simulink model "passive cell balancing"  (R2022a)
settings: Solver=VariableStepAuto  StartTime=0.0  StopTime=500  RelTol=1e-3
undefined symbols (not defined in the file): Ion, Lithium
libraries: spsIGBTLib x6, spsBatteryLib x4, spsSeriesRLCBranchLib x4, spsDCVoltageSourceLib x1, spsGroundLib x1, spsSeriesRLCLoadLib x1, spspowerguiLib x1
settings Model: Creator=my pc  LastModifiedBy=my pc

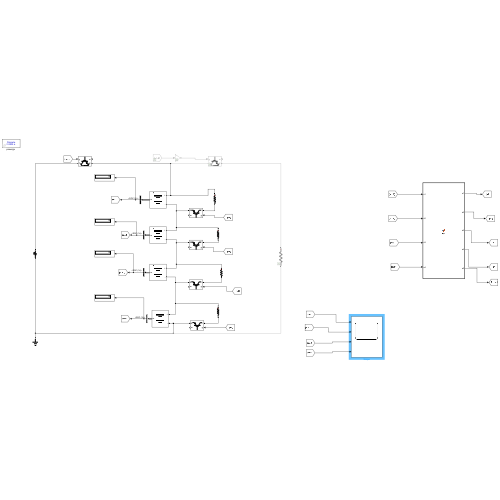
[thumbnail: Simulink's stored preview of the top-level diagram]
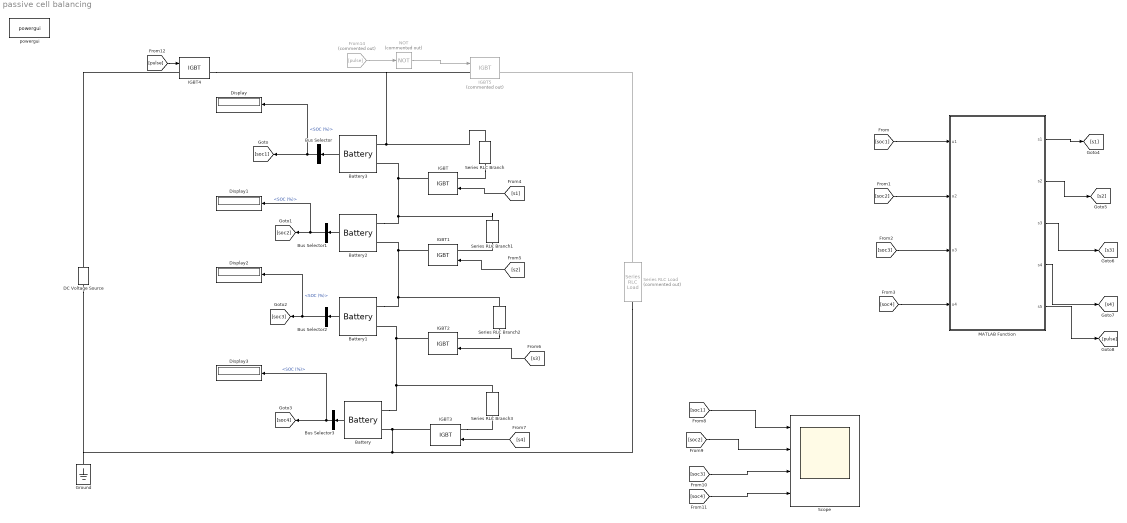
== system passive cell balancing ==
  Battery : spsBatteryLib/Battery  BatType=Lithium-Ion  ShowTempParam=off  ThermalPreset=no  ShowAgeParam=off  NomV=7.2  NomQ=5.4  SOC=19  Batt_Tr=30  PresetModel=on  MaxQ=5.4  MinV=5.4  FullV=8.3807  Dis_rate=2.3478  R=0.013333  Normal_OP=4.8835  expZone="[7.7788      0.2653]"  current=[6.5 13 32.5]  Units=Time  Tci=20  NomT=20  T2=-30  MaxQ2=4.8  FullV2=7.1  Normal_OP2=5.655  expZone2="[6.58           1]"  Rca=0.6  ti=2000  Dp=0  Neq0=0  Tsim=1e6  Ta1=25  Qeol=5.4*0.9  Reol=0.013333*1.2  Char_age=[2.3478, 3]  Dis_age=[2.3478, 10]  N1=1500  N2=10500  N3=1000  N4=1400  Ta2=45  N5=950
  Battery1 : spsBatteryLib/Battery  BatType=Lithium-Ion  ShowTempParam=off  ThermalPreset=no  ShowAgeParam=off  NomV=7.2  NomQ=5.4  SOC=21  Batt_Tr=30  PresetModel=on  MaxQ=5.4  MinV=5.4  FullV=8.3807  Dis_rate=2.3478  R=0.013333  Normal_OP=4.8835  expZone="[7.7788      0.2653]"  current=[6.5 13 32.5]  Units=Time  Tci=20  NomT=20  T2=-30  MaxQ2=4.8  FullV2=7.1  Normal_OP2=5.655  expZone2="[6.58           1]"  Rca=0.6  ti=2000  Dp=0  Neq0=0  Tsim=1e6  Ta1=25  Qeol=5.4*0.9  Reol=0.013333*1.2  Char_age=[2.3478, 3]  Dis_age=[2.3478, 10]  N1=1500  N2=10500  N3=1000  N4=1400  Ta2=45  N5=950
  Battery2 : spsBatteryLib/Battery  BatType=Lithium-Ion  ShowTempParam=off  ThermalPreset="3.3V  2.3Ah  (LiFePO4)"  ShowAgeParam=off  NomV=3.3  NomQ=2.3  SOC=25  Batt_Tr=30  PresetModel=off  MaxQ=2.3  MinV=2.475  FullV=3.748  Dis_rate=2.3  R=0.014  Normal_OP=2.25  expZone="[3.4788       0.113]"  current=[6.5 13 32.5]  Units=Time  Tci=25  NomT=25  T2=0  MaxQ2=2.208  FullV2=3.45  Normal_OP2=2.85  expZone2="[3.22       0.015]"  Rca=0.6  ti=1000  Dp=0  Neq0=5  Tsim=1e6  Ta1=25  Qeol=5.4*0.9  Reol=0.013333*1.2  Char_age=[2.3478, 3]  Dis_age=[2.3478, 10]  N1=1500  N2=10500  N3=1000  N4=1400  Ta2=45  N5=950
  Battery3 : spsBatteryLib/Battery  BatType=Lithium-Ion  ShowTempParam=off  ThermalPreset="3.3V  2.3Ah  (LiFePO4)"  ShowAgeParam=off  NomV=3.3  NomQ=2.3  SOC=22  Batt_Tr=30  PresetModel=off  MaxQ=2.3  MinV=2.475  FullV=3.748  Dis_rate=2.3  R=0.014  Normal_OP=2.25  expZone="[3.4788       0.113]"  current=[6.5 13 32.5]  Units=Time  Tci=20  NomT=25  T2=0  MaxQ2=2.208  FullV2=3.45  Normal_OP2=2.85  expZone2="[3.22       0.015]"  Rca=0.6  ti=1000  Dp=0  Neq0=0  Tsim=1e6  Ta1=25  Qeol=5.4*0.9  Reol=0.013333*1.2  Char_age=[2.3478, 3]  Dis_age=[2.3478, 10]  N1=1500  N2=10500  N3=1000  N4=1400  Ta2=45  N5=950
  Bus Selector{,1..3} (4 alike) : BusSelector  OutputSignals=SOC (%)
  DC Voltage Source : spsDCVoltageSourceLib/DC Voltage Source  Amplitude=12  Measurements=None
  Display{,1..3} (4 alike) : Display
  From14 : From  Commented=on  GotoTag=pulse
  Ground : spsGroundLib/Ground  LConnTagsString=a
  IGBT{,1..3} (4 alike) : spsIGBTLib/IGBT  Ron=0.001  Lon=0  Vf=1  Tf=1e-6  Tt=2e-6  IC=0  Rs=inf  Cs=inf  Measurements=on
  IGBT4 : spsIGBTLib/IGBT  Ron=0.001  Lon=0  Vf=1  Tf=1e-6  Tt=2e-6  IC=0  Rs=1e5  Cs=inf  Measurements=on
  IGBT5 : spsIGBTLib/IGBT  Commented=on  Ron=0.001  Lon=0  Vf=1  Tf=1e-6  Tt=2e-6  IC=0  Rs=1e5  Cs=inf  Measurements=on
  MATLAB Function : MATLAB Function  TreatAsAtomicUnit=on
  NOT : Logic  Commented=on  Operator=NOT  IconShape=distinctive  AllPortsSameDT=off  OutDataTypeStr=boolean
  Scope : Scope  NumInputPorts=4
  Series RLC Branch{,1..3} (4 alike) : spsSeriesRLCBranchLib/Series RLC Branch  LConnTagsString=__new0  RConnTagsString=__new0  BranchType=R  Resistance=0.5  Inductance=1e-3  SetiL0=off  InitialCurrent=0  Capacitance=1e-6  Setx0=off  InitialVoltage=0  Measurements=None
  Series RLC Load : spsSeriesRLCLoadLib/Series RLC Load  Commented=on  LConnTagsString=a  RConnTagsString=__new0  NominalVoltage=1000  NominalFrequency=60  ActivePower=10e5  InductivePower=0  CapacitivePower=0  Setx0=off  InitialVoltage=0  SetiL0=off  InitialCurrent=0  Measurements=None  LoadType=constant Z
  powergui : spspowerguiLib/powergui  Priority=1  SimulationMode=Discrete  SampleTime=0.0005  frequency=60  Iterations=50  frequencyindice=0  Pbase=100e6  ErrMax=1e-4  UnitsV=kV  UnitsW=MW  buscounter=0  FunctionMessages=off  echomessages=off  EnableUseOfTLC=off  CurrentSourceSwitches=off  DisableSnubberDevices=off  DisableRonSwitches=off  DisableVfSwitches=off  DisplayEquations=off  AutomaticDiscreteSolvers=off  SolverType=Tustin/Backward Euler (TBE)  Interpol=off  ExternalGateDelay=off  methode=off  Ts=100  x0status=blocks  SPID=on  SwTol=0  HookPort=off  NonlinearTolerance=1e-4  nMaxIteration=100  ContinueOnMaxIteration=off  RestoreLinks=warning  ResistiveCurrentMeasurement=off  Frange=[0:2:500]  Ylog=off  Xlog=on  ShowGrid=off  save=off  variable=ZData  structure=0  ZoomFFT=off  StartTime=0.0  cycles=1  DisplayStyle=1  fundamental=60  FreqAxis=off  MaxFrequency=1000  frequencyindicesteady=1  RmsSteady=1  display=off
  wires:
  Battery3/1 -> Bus Selector/1
  Bus Selector/1 -> [soc1], Display/1  "<SOC (%)>"
  Bus Selector1/1 -> Display1/1, [soc2]  "<SOC (%)>"
  Bus Selector2/1 -> Display2/1, [soc3]  "<SOC (%)>"
  Bus Selector3/1 -> [soc4], Display3/1  "<SOC (%)>"
  Battery/1 -> Bus Selector3/1
  Battery1/1 -> Bus Selector2/1
  Battery2/1 -> Bus Selector1/1
  [soc1] -> MATLAB Function/1(u1)
  [soc2] -> MATLAB Function/2(u2)
  [soc3] -> MATLAB Function/3(u3)
  [soc4] -> MATLAB Function/4(u4)
  MATLAB Function/1(s1) -> [s1]
  MATLAB Function/2(s2) -> [s2]
  MATLAB Function/3(s3) -> [s3]
  MATLAB Function/4(s4) -> [s4]
  [s1] -> IGBT/1
  [s2] -> IGBT1/1
  [s3] -> IGBT2/1
  [s4] -> IGBT3/1
  [soc1] -> Scope/1
  [soc2] -> Scope/2
  [soc3] -> Scope/3
  [soc4] -> Scope/4
  [pulse] -> IGBT4/1
  From14/1 -> NOT/1
  NOT/1 -> IGBT5/1
  MATLAB Function/5(s5) -> [pulse]
  connections:
  Battery1/LConn1 -- Series RLC Branch2/LConn1 -- IGBT1/RConn1 -- Battery2/LConn2
  Battery2/LConn1 -- Series RLC Branch1/LConn1 -- IGBT/RConn1 -- Battery3/LConn2
  Series RLC Branch/RConn1 -- IGBT/LConn1
  Series RLC Branch1/RConn1 -- IGBT1/LConn1
  Series RLC Branch2/RConn1 -- IGBT2/LConn1
  IGBT3/RConn1 -- Ground/LConn1 -- DC Voltage Source/LConn1 -- Series RLC Load/RConn1 -- Battery/LConn2
  IGBT3/LConn1 -- Series RLC Branch3/RConn1
  Series RLC Branch/LConn1 -- IGBT4/RConn1 -- IGBT5/LConn1 -- Battery3/LConn1
  Battery/LConn1 -- Series RLC Branch3/LConn1 -- Battery1/LConn2 -- IGBT2/RConn1
  DC Voltage Source/RConn1 -- IGBT4/LConn1
  Series RLC Load/LConn1 -- IGBT5/RConn1

== matlab function passive cell balancing/MATLAB Function ==
  data: u1 input; s1 output; u2 input; u3 input; u4 input; s2 output; s3 output; s4 output; s5 output
function [s1,s2,s3,s4,s5] = fcn(u1,u2,u3,u4)

u1=u1*1000;
u2=u2*1000;
u3=u3*1000;
u4=u4*1000;

u1=int32(u1);
u2=int32(u2);
u3=int32(u3);
u4=int32(u4);

a=[u1,u2,u3,u4];
data = min(a);

if (u1>data)
    s1=1;
else
    s1=0;
end

if (u2>data)
    s2=1;
else
    s2=0;
end

if (u3>data)
    s3=1;
else
    s3=0;
end

if (u4>data)
    s4=1;
else
    s4=0;
end
if(u1==u2 && u2==u3 && u3==u4)
    if(u1>80000)
    s5=0;
else s5=1;
    end
else
    s5=0;
end
